simulink library "motorlib"  (R2018a)
settings: Solver=VariableStepAuto  StartTime=0.0  StopTime=10.0  RelTol=1e-3
libraries: $bdroot x5, aerolibatmos2 x4
settings Model: Creator=mairon  LastModifiedBy=mairon

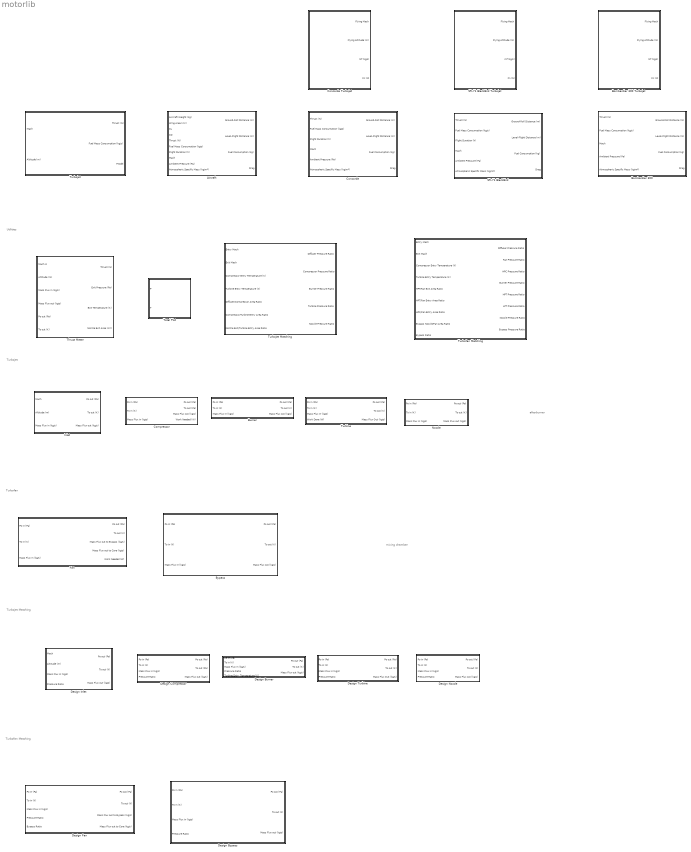
== system motorlib ==
  note: Turbofan Matching
  note: Utilities
  note: afterburner
  note: mixing chamber
  note: Turbofan
  note: Turbojet Matching
  note: Turbojet
  Aircraft : Subsystem
  Bombardier 300 : Subsystem  AncestorBlock=motorlib/Concorde
  Bombardier 300 Turbojet : Subsystem  AncestorBlock=motorlib/Concorde Turbojet
  Burner : Subsystem
  Bypass : Subsystem
  Compressor : Subsystem
  Concorde : Subsystem  AncestorBlock=motorlib/Aircraft
  Concorde Turbojet : Subsystem
  Design Burner : Subsystem  AncestorBlock=motorlib/Burner
  Design Bypass : Subsystem  AncestorBlock=motorlib/Bypass
  Design Compressor : Subsystem  AncestorBlock=motorlib/Compressor
  Design Fan : Subsystem  AncestorBlock=motorlib/Fan
  Design Inlet : Subsystem  AncestorBlock=motorlib/Inlet
  Design Nozzle : Subsystem  AncestorBlock=motorlib/Nozzle
  Design Turbine : Subsystem  AncestorBlock=motorlib/Turbine
  Fan : Subsystem
  Inlet : Subsystem
  Nozzle : Subsystem
  SR-71 BlackBird : Subsystem  AncestorBlock=motorlib/Concorde
  SR-71 BlackBird Turbojet : Subsystem  AncestorBlock=motorlib/Concorde Turbojet
  Thrust Meter : Subsystem
  Total Plot : MATLAB Function  TreatAsAtomicUnit=on
  Turbine : Subsystem
  Turbofan Matching : Subsystem  AncestorBlock=motorlib/Turbojet Matching
  Turbojet : Subsystem
  Turbojet Matching : Subsystem

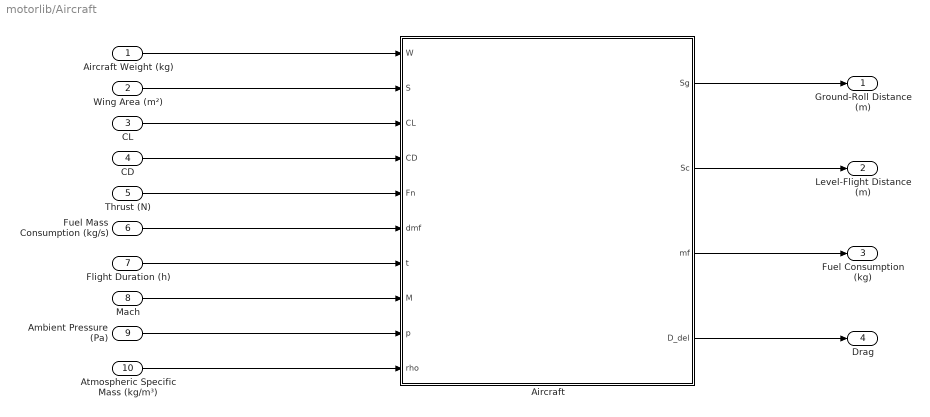
== system motorlib/Aircraft ==
  Aircraft Weight (kg) : Inport
  Wing Area (m²) : Inport  Port=2
  CL : Inport  Port=3
  CD : Inport  Port=4
  Thrust (N) : Inport  Port=5
  Fuel Mass Consumption (kg/s) : Inport  Port=6
  Flight Duration (h) : Inport  Port=7
  Mach : Inport  Port=8
  Ambient Pressure (Pa) : Inport  Port=9
  Atmospheric Specific Mass (kg/m³) : Inport  Port=10
  Aircraft : MATLAB Function  TreatAsAtomicUnit=on
  Ground-Roll Distance (m) : Outport
  Level-Flight Distance (m) : Outport  Port=2
  Fuel Consumption (kg) : Outport  Port=3
  Drag : Outport  Port=4
  wires:
  Aircraft/1(Sg) -> Ground-Roll Distance (m)/1
  Aircraft Weight (kg)/1 -> Aircraft/1(W)
  CD/1 -> Aircraft/4(CD)
  Wing Area (m²)/1 -> Aircraft/2(S)
  Aircraft/2(Sc) -> Level-Flight Distance (m)/1
  Ambient Pressure (Pa)/1 -> Aircraft/9(p)
  Fuel Mass Consumption (kg/s)/1 -> Aircraft/6(dmf)
  Aircraft/3(mf) -> Fuel Consumption (kg)/1
  Mach/1 -> Aircraft/8(M)
  CL/1 -> Aircraft/3(CL)
  Thrust (N)/1 -> Aircraft/5(Fn)
  Flight Duration (h)/1 -> Aircraft/7(t)
  Atmospheric Specific Mass (kg/m³)/1 -> Aircraft/10(rho)
  Aircraft/4(D_del) -> Drag/1

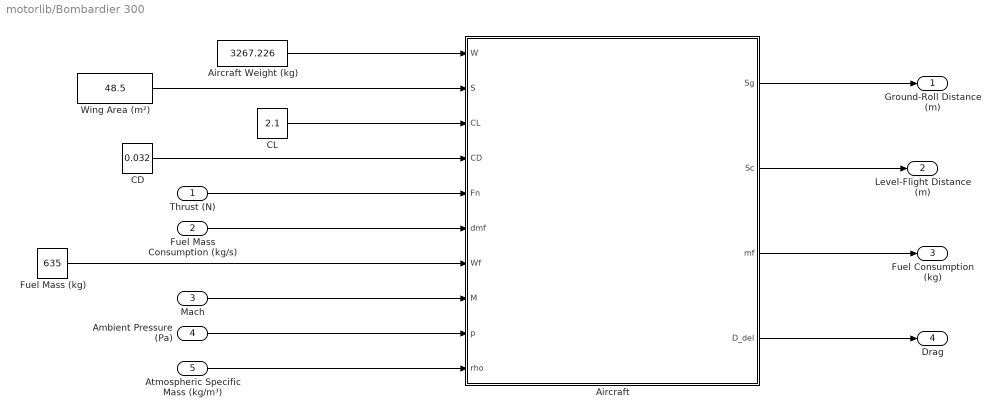
== system motorlib/Bombardier 300 ==
  Thrust (N) : Inport
  Fuel Mass Consumption (kg/s) : Inport  Port=2
  Mach : Inport  Port=3
  Ambient Pressure (Pa) : Inport  Port=4
  Atmospheric Specific Mass (kg/m³) : Inport  Port=5
  Aircraft : MATLAB Function  TreatAsAtomicUnit=on
  Aircraft Weight (kg) : Constant  Value=3267.226
  CD : Constant  Value=0.032
  CL : Constant  Value=2.1
  Fuel Mass (kg) : Constant  Value=635
  Wing Area (m²) : Constant  Value=48.5
  Ground-Roll Distance (m) : Outport
  Level-Flight Distance (m) : Outport  Port=2
  Fuel Consumption (kg) : Outport  Port=3
  Drag : Outport  Port=4
  wires:
  Aircraft/1(Sg) -> Ground-Roll Distance (m)/1
  Aircraft/2(Sc) -> Level-Flight Distance (m)/1
  Ambient Pressure (Pa)/1 -> Aircraft/9(p)
  Fuel Mass Consumption (kg/s)/1 -> Aircraft/6(dmf)
  Aircraft/3(mf) -> Fuel Consumption (kg)/1
  Mach/1 -> Aircraft/8(M)
  Thrust (N)/1 -> Aircraft/5(Fn)
  Fuel Mass (kg)/1 -> Aircraft/7(Wf)
  Atmospheric Specific Mass (kg/m³)/1 -> Aircraft/10(rho)
  Wing Area (m²)/1 -> Aircraft/2(S)
  CD/1 -> Aircraft/4(CD)
  CL/1 -> Aircraft/3(CL)
  Aircraft Weight (kg)/1 -> Aircraft/1(W)
  Aircraft/4(D_del) -> Drag/1

== system motorlib/Bombardier 300 Turbojet ==
  Altitude (m) : Constant  Value=9100
  Mach : Constant  Value=0.63
  Mass Fuel Consumption (kg/s) : Constant  Value=0.100
  Thrust (N) : Constant  Value=9319*2
  Flying Mach : Outport
  Flying Altitude (m) : Outport  Port=2
  mf (kg/s) : Outport  Port=3
  Fn (N) : Outport  Port=4
  wires:
  Altitude (m)/1 -> Flying Altitude (m)/1
  Mass Fuel Consumption (kg/s)/1 -> mf (kg/s)/1
  Mach/1 -> Flying Mach/1
  Thrust (N)/1 -> Fn (N)/1

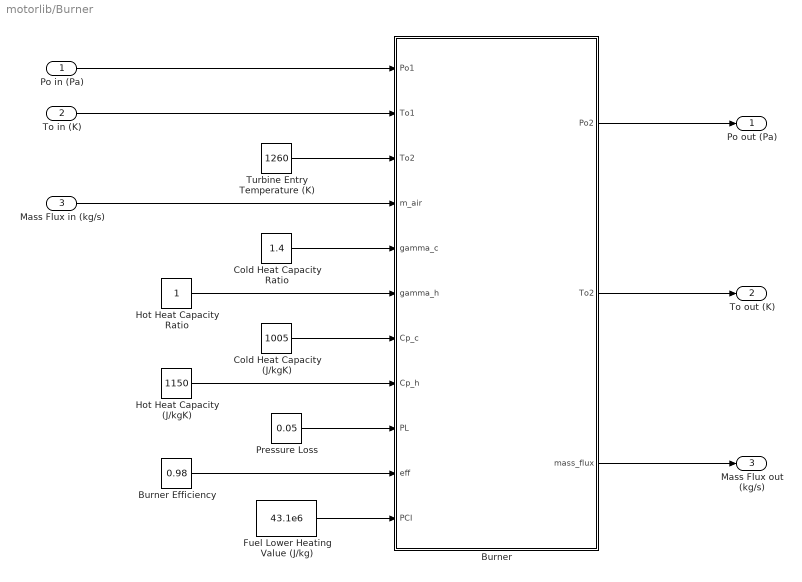
== system motorlib/Burner ==
  Po in (Pa) : Inport
  To in (K) : Inport  Port=2
  Mass Flux in (kg/s) : Inport  Port=3
  Burner : MATLAB Function  TreatAsAtomicUnit=on
  Burner Efficiency : Constant  Value=0.98
  Cold Heat Capacity (J/kgK) : Constant  Value=1005
  Cold Heat Capacity Ratio : Constant  Value=1.4
  Fuel Lower Heating Value (J/kg) : Constant  Value=43.1e6
  Hot Heat Capacity (J/kgK) : Constant  Value=1150
  Hot Heat Capacity Ratio : Constant
  Pressure Loss : Constant  Value=0.05
  Turbine Entry Temperature (K) : Constant  Value=1260
  Po out (Pa) : Outport
  To out (K) : Outport  Port=2
  Mass Flux out (kg/s) : Outport  Port=3
  wires:
  Cold Heat Capacity (J/kgK)/1 -> Burner/7(Cp_c)
  Pressure Loss/1 -> Burner/9(PL)
  Po in (Pa)/1 -> Burner/1(Po1)
  Burner/2(To2) -> To out (K)/1
  Turbine Entry Temperature (K)/1 -> Burner/3("To2 ")
  Hot Heat Capacity (J/kgK)/1 -> Burner/8(Cp_h)
  To in (K)/1 -> Burner/2(To1)
  Burner/3(mass_flux) -> Mass Flux out (kg/s)/1
  Fuel Lower Heating Value (J/kg)/1 -> Burner/11(PCI)
  Cold Heat Capacity Ratio/1 -> Burner/5(gamma_c)
  Mass Flux in (kg/s)/1 -> Burner/4(m_air)
  Burner/1(Po2) -> Po out (Pa)/1
  Burner Efficiency/1 -> Burner/10(eff)
  Hot Heat Capacity Ratio/1 -> Burner/6(gamma_h)

== system motorlib/Bypass ==
  Po in (Pa) : Inport
  To in (K) : Inport  Port=2
  Mass Flux in (kg/s) : Inport  Port=3
  Bypass : MATLAB Function  TreatAsAtomicUnit=on
  Heat Capacity Ratio : Constant  Value=1.4
  Pressure Loss : Constant  Value=0.05
  Po out (Pa) : Outport
  To out (K) : Outport  Port=2
  Mass Flux out (kg/s) : Outport  Port=3
  wires:
  Bypass/2(To2) -> To out (K)/1
  Bypass/1(Po2) -> Po out (Pa)/1
  Mass Flux in (kg/s)/1 -> Bypass/3("mass_flux ")
  To in (K)/1 -> Bypass/2(To1)
  Po in (Pa)/1 -> Bypass/1(Po1)
  Pressure Loss/1 -> Bypass/5(PL)
  Bypass/3(mass_flux) -> Mass Flux out (kg/s)/1
  Heat Capacity Ratio/1 -> Bypass/4(gamma)

== system motorlib/Compressor ==
  Po in (Pa) : Inport
  To in (K) : Inport  Port=2
  Mass Flux in (kg/s) : Inport  Port=3
  Compressor : MATLAB Function  TreatAsAtomicUnit=on
  Compressor Eficiency : Constant  Value=0.85
  Heat Capacity (J/kgK) : Constant  Value=1005
  Heat Capacity Ratio : Constant  Value=1.4
  Pressure Ratio : Constant  Value=13.5
  Po out (Pa) : Outport
  To out (Pa) : Outport  Port=2
  Mass Flux out (kg/s) : Outport  Port=3
  Work Needed (W) : Outport  Port=4
  wires:
  Mass Flux in (kg/s)/1 -> Compressor/3(m_air)
  Compressor/4(W) -> Work Needed (W)/1
  Compressor/2(To2) -> To out (Pa)/1
  Po in (Pa)/1 -> Compressor/1(Po1)
  Compressor/1(Po2) -> Po out (Pa)/1
  To in (K)/1 -> Compressor/2(To1)
  Compressor/3(mass_flux) -> Mass Flux out (kg/s)/1
  Heat Capacity Ratio/1 -> Compressor/4(gamma)
  Heat Capacity (J/kgK)/1 -> Compressor/5(Cp)
  Pressure Ratio/1 -> Compressor/6(PR)
  Compressor Eficiency/1 -> Compressor/7(eff)

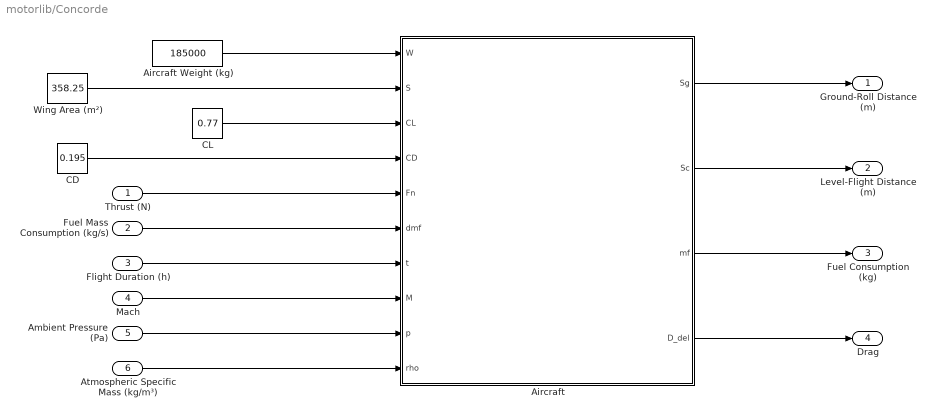
== system motorlib/Concorde ==
  Thrust (N) : Inport
  Fuel Mass Consumption (kg/s) : Inport  Port=2
  Flight Duration (h) : Inport  Port=3
  Mach : Inport  Port=4
  Ambient Pressure (Pa) : Inport  Port=5
  Atmospheric Specific Mass (kg/m³) : Inport  Port=6
  Aircraft : MATLAB Function  TreatAsAtomicUnit=on
  Aircraft Weight (kg) : Constant  Value=185000
  CD : Constant  Value=0.195
  CL : Constant  Value=0.77
  Wing Area (m²) : Constant  Value=358.25
  Ground-Roll Distance (m) : Outport
  Level-Flight Distance (m) : Outport  Port=2
  Fuel Consumption (kg) : Outport  Port=3
  Drag : Outport  Port=4
  wires:
  Aircraft/1(Sg) -> Ground-Roll Distance (m)/1
  Aircraft/2(Sc) -> Level-Flight Distance (m)/1
  Ambient Pressure (Pa)/1 -> Aircraft/9(p)
  Fuel Mass Consumption (kg/s)/1 -> Aircraft/6(dmf)
  Aircraft/3(mf) -> Fuel Consumption (kg)/1
  Mach/1 -> Aircraft/8(M)
  Thrust (N)/1 -> Aircraft/5(Fn)
  Flight Duration (h)/1 -> Aircraft/7(t)
  Atmospheric Specific Mass (kg/m³)/1 -> Aircraft/10(rho)
  Wing Area (m²)/1 -> Aircraft/2(S)
  CD/1 -> Aircraft/4(CD)
  CL/1 -> Aircraft/3(CL)
  Aircraft Weight (kg)/1 -> Aircraft/1(W)
  Aircraft/4(D_del) -> Drag/1

== system motorlib/Concorde Turbojet ==
  Altitude (m) : Constant  Value=18000
  Mach : Constant  Value=2
  Mass Fuel Consumption (kg/s) : Constant  Value=5.699
  Thrust (N) : Constant  Value=17233*4
  Flying Mach : Outport
  Flying Altitude (m) : Outport  Port=2
  mf (kg/s) : Outport  Port=3
  Fn (N) : Outport  Port=4
  wires:
  Thrust (N)/1 -> Fn (N)/1
  Mach/1 -> Flying Mach/1
  Mass Fuel Consumption (kg/s)/1 -> mf (kg/s)/1
  Altitude (m)/1 -> Flying Altitude (m)/1

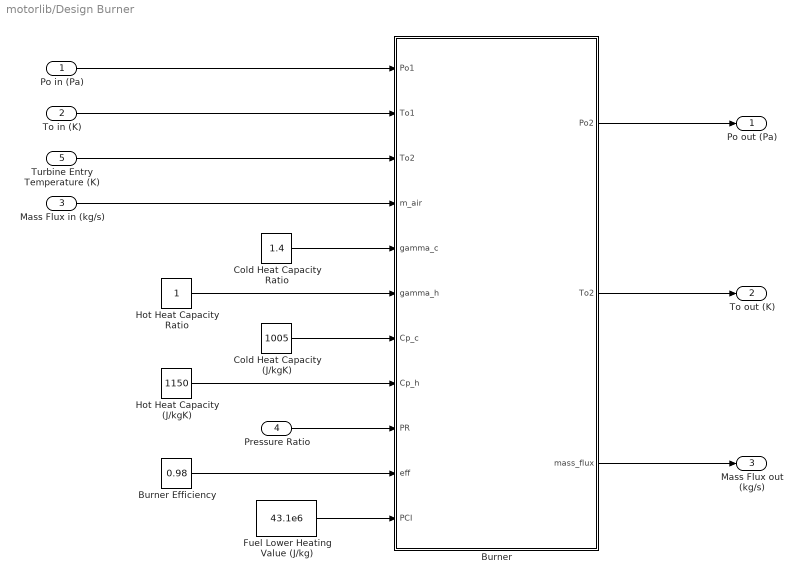
== system motorlib/Design Burner ==
  Po in (Pa) : Inport
  To in (K) : Inport  Port=2
  Mass Flux in (kg/s) : Inport  Port=3
  Pressure Ratio : Inport  Port=4
  Turbine Entry Temperature (K) : Inport  Port=5
  Burner : MATLAB Function  TreatAsAtomicUnit=on
  Burner Efficiency : Constant  Value=0.98
  Cold Heat Capacity (J/kgK) : Constant  Value=1005
  Cold Heat Capacity Ratio : Constant  Value=1.4
  Fuel Lower Heating Value (J/kg) : Constant  Value=43.1e6
  Hot Heat Capacity (J/kgK) : Constant  Value=1150
  Hot Heat Capacity Ratio : Constant
  Po out (Pa) : Outport
  To out (K) : Outport  Port=2
  Mass Flux out (kg/s) : Outport  Port=3
  wires:
  Hot Heat Capacity Ratio/1 -> Burner/6(gamma_h)
  Burner Efficiency/1 -> Burner/10(eff)
  Burner/1(Po2) -> Po out (Pa)/1
  Mass Flux in (kg/s)/1 -> Burner/4(m_air)
  Cold Heat Capacity Ratio/1 -> Burner/5(gamma_c)
  Fuel Lower Heating Value (J/kg)/1 -> Burner/11(PCI)
  Burner/3(mass_flux) -> Mass Flux out (kg/s)/1
  To in (K)/1 -> Burner/2(To1)
  Hot Heat Capacity (J/kgK)/1 -> Burner/8(Cp_h)
  Turbine Entry Temperature (K)/1 -> Burner/3("To2 ")
  Burner/2(To2) -> To out (K)/1
  Po in (Pa)/1 -> Burner/1(Po1)
  Pressure Ratio/1 -> Burner/9(PR)
  Cold Heat Capacity (J/kgK)/1 -> Burner/7(Cp_c)

== system motorlib/Design Bypass ==
  Po in (Pa) : Inport
  To in (K) : Inport  Port=2
  Mass Flux in (kg/s) : Inport  Port=3
  Pressure Ratio : Inport  Port=4
  Bypass : MATLAB Function  TreatAsAtomicUnit=on
  Heat Capacity Ratio : Constant  Value=1.4
  Po out (Pa) : Outport
  To out (K) : Outport  Port=2
  Mass Flux out (kg/s) : Outport  Port=3
  wires:
  Bypass/2(To2) -> To out (K)/1
  Bypass/1(Po2) -> Po out (Pa)/1
  Mass Flux in (kg/s)/1 -> Bypass/3("mass_flux ")
  To in (K)/1 -> Bypass/2(To1)
  Po in (Pa)/1 -> Bypass/1(Po1)
  Pressure Ratio/1 -> Bypass/5(PR)
  Bypass/3(mass_flux) -> Mass Flux out (kg/s)/1
  Heat Capacity Ratio/1 -> Bypass/4(gamma)

== system motorlib/Design Compressor ==
  Po in (Pa) : Inport
  To in (K) : Inport  Port=2
  Mass Flux in (kg/s) : Inport  Port=3
  Pressure Ratio : Inport  Port=4
  Compressor : MATLAB Function  TreatAsAtomicUnit=on
  Compressor Eficiency : Constant  Value=0.85
  Heat Capacity (J/kgK) : Constant  Value=1005
  Heat Capacity Ratio : Constant  Value=1.4
  Po out (Pa) : Outport
  To out (Pa) : Outport  Port=2
  Mass Flux out (kg/s) : Outport  Port=3
  wires:
  Compressor Eficiency/1 -> Compressor/7(eff)
  Pressure Ratio/1 -> Compressor/6(PR)
  Heat Capacity (J/kgK)/1 -> Compressor/5(Cp)
  Heat Capacity Ratio/1 -> Compressor/4(gamma)
  Compressor/3(mass_flux) -> Mass Flux out (kg/s)/1
  To in (K)/1 -> Compressor/2(To1)
  Compressor/1(Po2) -> Po out (Pa)/1
  Po in (Pa)/1 -> Compressor/1(Po1)
  Compressor/2(To2) -> To out (Pa)/1
  Mass Flux in (kg/s)/1 -> Compressor/3(m_air)

== system motorlib/Design Fan ==
  Po in (Pa) : Inport
  To in (K) : Inport  Port=2
  Mass Flux in (kg/s) : Inport  Port=3
  Pressure Ratio : Inport  Port=4
  Bypass Ratio : Inport  Port=5
  Efficiency : Constant  Value=0.84
  Fan : MATLAB Function  TreatAsAtomicUnit=on
  Heat Capacity (J/kgK) : Constant  Value=1005
  Heat Capacity Ratio : Constant  Value=1.4
  Po out (Pa) : Outport
  To out (K) : Outport  Port=2
  Mass Flux out to Bypass (kg/s) : Outport  Port=3
  Mass Flux out to Core (kg/s) : Outport  Port=4
  wires:
  Fan/1(Po2) -> Po out (Pa)/1
  Po in (Pa)/1 -> Fan/1(Po1)
  Fan/2(To2) -> To out (K)/1
  Heat Capacity (J/kgK)/1 -> Fan/5(Cp)
  Fan/4(mass_flux_core) -> Mass Flux out to Core (kg/s)/1
  Fan/3(mass_flux_bp) -> Mass Flux out to Bypass (kg/s)/1
  Efficiency/1 -> Fan/7(eff)
  Heat Capacity Ratio/1 -> Fan/4(gamma)
  To in (K)/1 -> Fan/2(To1)
  Bypass Ratio/1 -> Fan/8(B)
  Mass Flux in (kg/s)/1 -> Fan/3(mass_flux)
  Pressure Ratio/1 -> Fan/6(PR)

== system motorlib/Design Inlet ==
  Mach : Inport
  Altitude (m) : Inport  Port=2
  Mass Flux in (kg/s) : Inport  Port=3
  Pressure Ratio : Inport  Port=4
  Heat Capacity Ratio : Constant  Value=1.4
  ISA Atmosphere Model : aerolibatmos2/ISA Atmosphere Model  custom=off  g=9.80665  gamma=1.4  R=287.0531  L=0.0065  h_trop=11000  h_strat=20000  rho0=1.225  P0=101325  T0=288.15  h0=0
      settings: SourceProductName=Aerospace Blockset
  Inlet : MATLAB Function  TreatAsAtomicUnit=on
  Po out (Pa) : Outport
  To out (K) : Outport  Port=2
  Mass Flux out (kg/s) : Outport  Port=3
  wires:
  Heat Capacity Ratio/1 -> Inlet/4(gamma)
  Inlet/3(mass_flux) -> Mass Flux out (kg/s)/1
  Mass Flux in (kg/s)/1 -> Inlet/6(m_air)
  Altitude (m)/1 -> ISA Atmosphere Model/1
  ISA Atmosphere Model/3 -> Inlet/2(P)
  Pressure Ratio/1 -> Inlet/5(PR)
  Inlet/1(Po) -> Po out (Pa)/1
  ISA Atmosphere Model/1 -> Inlet/3(T)
  Mach/1 -> Inlet/1(Mach)
  Inlet/2(To) -> To out (K)/1

== system motorlib/Design Nozzle ==
  Po in (Pa) : Inport
  To in (K) : Inport  Port=2
  Mass Flux in (kg/s) : Inport  Port=3
  Pressure Ratio : Inport  Port=4
  Hot Heat Capacity Ratio : Constant  Value=1.333
  Nozzle : MATLAB Function  TreatAsAtomicUnit=on
  Po out (Pa) : Outport
  To out (K) : Outport  Port=2
  Mass Flux out (kg/s) : Outport  Port=3
  wires:
  Hot Heat Capacity Ratio/1 -> Nozzle/4(gamma)
  Pressure Ratio/1 -> Nozzle/5(PR)
  Nozzle/3(mass_flux) -> Mass Flux out (kg/s)/1
  Nozzle/1(Po2) -> Po out (Pa)/1
  Mass Flux in (kg/s)/1 -> Nozzle/3("mass_flux ")
  To in (K)/1 -> Nozzle/2(To1)
  Nozzle/2(To2) -> To out (K)/1
  Po in (Pa)/1 -> Nozzle/1(Po1)

== system motorlib/Design Turbine ==
  Po in (Pa) : Inport
  To in (K) : Inport  Port=2
  Mass Flux in (kg/s) : Inport  Port=3
  Pressure Ratio : Inport  Port=4
  Efficiency : Constant
  Hot Heat Capacity Ratio : Constant  Value=1.333
  Turbine : MATLAB Function  TreatAsAtomicUnit=on
  Po out (Pa) : Outport
  To out (K) : Outport  Port=2
  Mass Flux Out (kg/s) : Outport  Port=3
  wires:
  Mass Flux in (kg/s)/1 -> Turbine/3("mass_flux ")
  Po in (Pa)/1 -> Turbine/1(Po1)
  Turbine/3(mass_flux) -> Mass Flux Out (kg/s)/1
  Hot Heat Capacity Ratio/1 -> Turbine/5(gamma)
  Turbine/1(Po2) -> Po out (Pa)/1
  Pressure Ratio/1 -> Turbine/4(PR)
  To in (K)/1 -> Turbine/2(To1)
  Turbine/2(To2) -> To out (K)/1
  Efficiency/1 -> Turbine/6(eff)

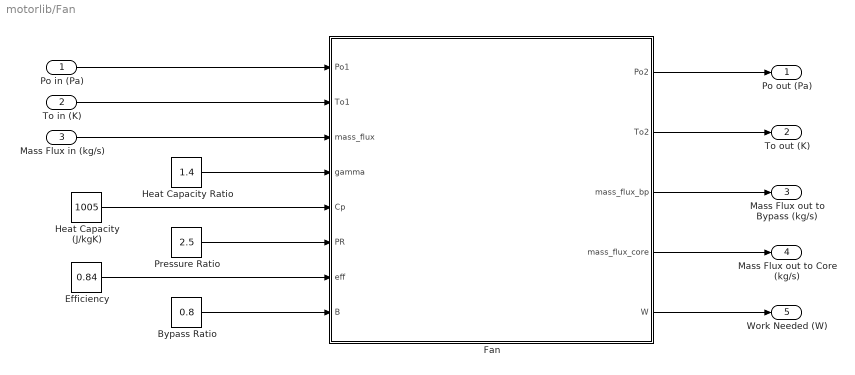
== system motorlib/Fan ==
  Po in (Pa) : Inport
  To in (K) : Inport  Port=2
  Mass Flux in (kg/s) : Inport  Port=3
  Bypass Ratio : Constant  Value=0.8
  Efficiency : Constant  Value=0.84
  Fan : MATLAB Function  TreatAsAtomicUnit=on
  Heat Capacity (J/kgK) : Constant  Value=1005
  Heat Capacity Ratio : Constant  Value=1.4
  Pressure Ratio : Constant  Value=2.5
  Po out (Pa) : Outport
  To out (K) : Outport  Port=2
  Mass Flux out to Bypass (kg/s) : Outport  Port=3
  Mass Flux out to Core (kg/s) : Outport  Port=4
  Work Needed (W) : Outport  Port=5
  wires:
  Fan/1(Po2) -> Po out (Pa)/1
  Po in (Pa)/1 -> Fan/1(Po1)
  Fan/2(To2) -> To out (K)/1
  Heat Capacity (J/kgK)/1 -> Fan/5(Cp)
  Fan/4(mass_flux_core) -> Mass Flux out to Core (kg/s)/1
  Fan/5(W) -> Work Needed (W)/1
  Fan/3(mass_flux_bp) -> Mass Flux out to Bypass (kg/s)/1
  Efficiency/1 -> Fan/7(eff)
  Heat Capacity Ratio/1 -> Fan/4(gamma)
  To in (K)/1 -> Fan/2(To1)
  Bypass Ratio/1 -> Fan/8(B)
  Mass Flux in (kg/s)/1 -> Fan/3(mass_flux)
  Pressure Ratio/1 -> Fan/6(PR)

== system motorlib/Inlet ==
  Mach : Inport
  Altitude (m) : Inport  Port=2
  Mass Flux in (kg/s) : Inport  Port=3
  Heat Capacity Ratio : Constant  Value=1.4
  ISA Atmosphere Model : aerolibatmos2/ISA Atmosphere Model  custom=off  g=9.80665  gamma=1.4  R=287.0531  L=0.0065  h_trop=11000  h_strat=20000  rho0=1.225  P0=101325  T0=288.15  h0=0
      settings: SourceProductName=Aerospace Blockset
  Inlet : MATLAB Function  TreatAsAtomicUnit=on
  Pressure Loss : Constant  Value=0
  Po out (Pa) : Outport
  To out (K) : Outport  Port=2
  Mass Flux out (kg/s) : Outport  Port=3
  wires:
  Inlet/2(To) -> To out (K)/1
  Mach/1 -> Inlet/1(Mach)
  ISA Atmosphere Model/1 -> Inlet/3(T)
  Inlet/1(Po) -> Po out (Pa)/1
  Pressure Loss/1 -> Inlet/5(PL)
  ISA Atmosphere Model/3 -> Inlet/2(P)
  Altitude (m)/1 -> ISA Atmosphere Model/1
  Mass Flux in (kg/s)/1 -> Inlet/6(m_air)
  Inlet/3(mass_flux) -> Mass Flux out (kg/s)/1
  Heat Capacity Ratio/1 -> Inlet/4(gamma)

== system motorlib/Nozzle ==
  Po in (Pa) : Inport
  To in (K) : Inport  Port=2
  Mass Flux in (kg/s) : Inport  Port=3
  Hot Heat Capacity Ratio : Constant  Value=1.333
  Nozzle : MATLAB Function  TreatAsAtomicUnit=on
  Pressure Loss : Constant  Value=0.02
  Po out (Pa) : Outport
  To out (K) : Outport  Port=2
  Mass Flux out (kg/s) : Outport  Port=3
  wires:
  Po in (Pa)/1 -> Nozzle/1(Po1)
  Nozzle/2(To2) -> To out (K)/1
  To in (K)/1 -> Nozzle/2(To1)
  Mass Flux in (kg/s)/1 -> Nozzle/3("mass_flux ")
  Nozzle/1(Po2) -> Po out (Pa)/1
  Nozzle/3(mass_flux) -> Mass Flux out (kg/s)/1
  Pressure Loss/1 -> Nozzle/5(PL)
  Hot Heat Capacity Ratio/1 -> Nozzle/4(gamma)

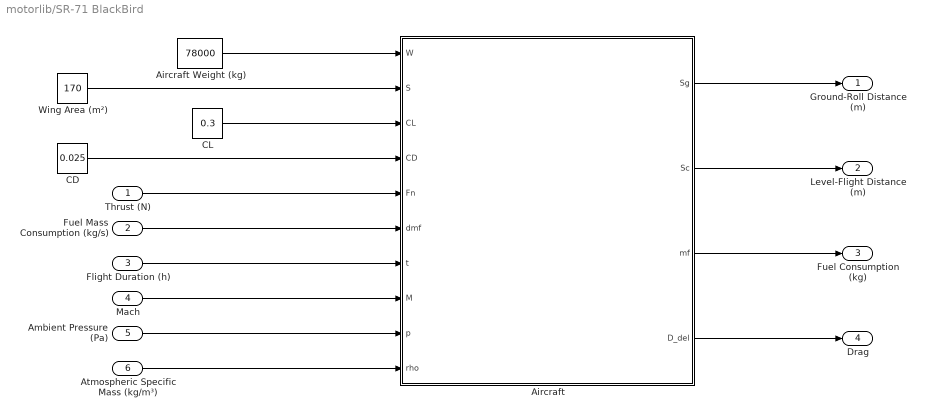
== system motorlib/SR-71 BlackBird ==
  Thrust (N) : Inport
  Fuel Mass Consumption (kg/s) : Inport  Port=2
  Flight Duration (h) : Inport  Port=3
  Mach : Inport  Port=4
  Ambient Pressure (Pa) : Inport  Port=5
  Atmospheric Specific Mass (kg/m³) : Inport  Port=6
  Aircraft : MATLAB Function  TreatAsAtomicUnit=on
  Aircraft Weight (kg) : Constant  Value=78000
  CD : Constant  Value=0.025
  CL : Constant  Value=0.3
  Wing Area (m²) : Constant  Value=170
  Ground-Roll Distance (m) : Outport
  Level-Flight Distance (m) : Outport  Port=2
  Fuel Consumption (kg) : Outport  Port=3
  Drag : Outport  Port=4
  wires:
  Aircraft/1(Sg) -> Ground-Roll Distance (m)/1
  Aircraft/2(Sc) -> Level-Flight Distance (m)/1
  Ambient Pressure (Pa)/1 -> Aircraft/9(p)
  Fuel Mass Consumption (kg/s)/1 -> Aircraft/6(dmf)
  Aircraft/3(mf) -> Fuel Consumption (kg)/1
  Mach/1 -> Aircraft/8(M)
  Thrust (N)/1 -> Aircraft/5(Fn)
  Flight Duration (h)/1 -> Aircraft/7(t)
  Atmospheric Specific Mass (kg/m³)/1 -> Aircraft/10(rho)
  Wing Area (m²)/1 -> Aircraft/2(S)
  CD/1 -> Aircraft/4(CD)
  CL/1 -> Aircraft/3(CL)
  Aircraft Weight (kg)/1 -> Aircraft/1(W)
  Aircraft/4(D_del) -> Drag/1

== system motorlib/SR-71 BlackBird Turbojet ==
  Altitude (m) : Constant  Value=25910
  Mach : Constant  Value=3.17
  Mass Fuel Consumption (kg/s) : Constant  Value=4.17
  Thrust (N) : Constant  Value=151000*2
  Flying Mach : Outport
  Flying Altitude (m) : Outport  Port=2
  mf (kg/s) : Outport  Port=3
  Fn (N) : Outport  Port=4
  wires:
  Thrust (N)/1 -> Fn (N)/1
  Mach/1 -> Flying Mach/1
  Mass Fuel Consumption (kg/s)/1 -> mf (kg/s)/1
  Altitude (m)/1 -> Flying Altitude (m)/1

== system motorlib/Thrust Meter ==
  Mach in : Inport
  Altitude (m) : Inport  Port=2
  Mass Flux in (kg/s) : Inport  Port=3
  Mass Flux out (kg/s) : Inport  Port=4
  Po out (Pa) : Inport  Port=5
  To out (K) : Inport  Port=6
  Hot Heat Capacity Ratio : Constant  Value=1.333
  ISA Atmosphere Model1 : aerolibatmos2/ISA Atmosphere Model  custom=off  g=9.80665  gamma=1.4  R=287.0531  L=0.0065  h_trop=11000  h_strat=20000  rho0=1.225  P0=101325  T0=288.15  h0=0
      settings: SourceProductName=Aerospace Blockset
  Thrust : MATLAB Function  TreatAsAtomicUnit=on
  Thrust (N) : Outport
  Exit Pressure (Pa) : Outport  Port=2
  Exit Temperature (K) : Outport  Port=3
  Nozzle Exit Area (m²) : Outport  Port=4
  wires:
  ISA Atmosphere Model1/1 -> Thrust/4(Tatm)
  ISA Atmosphere Model1/3 -> Thrust/3(Patm)
  Altitude (m)/1 -> ISA Atmosphere Model1/1
  Mach in/1 -> Thrust/1(Mo)
  ISA Atmosphere Model1/2 -> Thrust/2(a)
  Mass Flux in (kg/s)/1 -> Thrust/5(mass_flux_0)
  Mass Flux out (kg/s)/1 -> Thrust/6(mass_flux)
  Hot Heat Capacity Ratio/1 -> Thrust/9(gamma_h)
  Po out (Pa)/1 -> Thrust/7(Po2)
  To out (K)/1 -> Thrust/8(To2)
  Thrust/2(Pe) -> Exit Pressure (Pa)/1
  Thrust/3(Te) -> Exit Temperature (K)/1
  Thrust/1(FN) -> Thrust (N)/1
  Thrust/4(Ae) -> Nozzle Exit Area (m²)/1

== system motorlib/Turbine ==
  Po in (Pa) : Inport
  To in (K) : Inport  Port=2
  Mass Flux in (kg/s) : Inport  Port=3
  Work Done (W) : Inport  Port=4
  Hot Heat Capacity (J/kgK) : Constant  Value=1150
  Hot Heat Capacity Ratio : Constant  Value=1.333
  Turbine : MATLAB Function  TreatAsAtomicUnit=on
  Turbine Efficiency : Constant  Value=0.92
  Po out (Pa) : Outport
  To out (K) : Outport  Port=2
  Mass Flux Out (kg/s) : Outport  Port=3
  wires:
  Turbine/2(To2) -> To out (K)/1
  To in (K)/1 -> Turbine/2(To1)
  Work Done (W)/1 -> Turbine/4(W)
  Turbine/1(Po2) -> Po out (Pa)/1
  Hot Heat Capacity (J/kgK)/1 -> Turbine/6(Cp_h)
  Hot Heat Capacity Ratio/1 -> Turbine/5(gamma_h)
  Turbine/3(mass_flux) -> Mass Flux Out (kg/s)/1
  Turbine Efficiency/1 -> Turbine/7(eff)
  Po in (Pa)/1 -> Turbine/1(Po1)
  Mass Flux in (kg/s)/1 -> Turbine/3("mass_flux ")

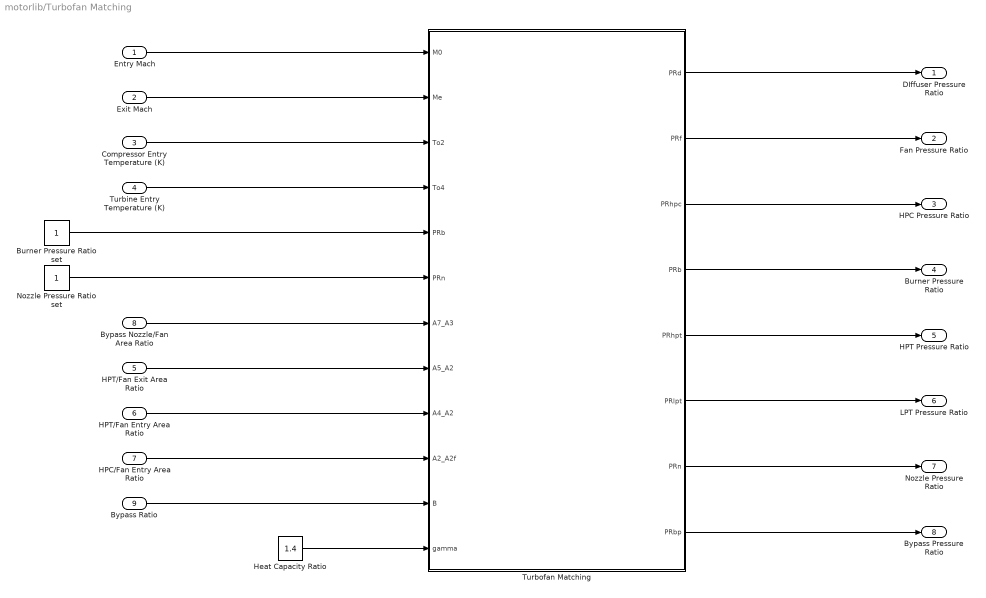
== system motorlib/Turbofan Matching ==
  Entry Mach : Inport
  Exit Mach : Inport  Port=2
  Compressor Entry Temperature (K) : Inport  Port=3
  Turbine Entry Temperature (K) : Inport  Port=4
  HPT/Fan Exit Area Ratio : Inport  Port=5
  HPT/Fan Entry Area Ratio : Inport  Port=6
  HPC/Fan Entry Area Ratio : Inport  Port=7
  Bypass Nozzle/Fan Area Ratio : Inport  Port=8
  "Bypass Ratio " : Inport  Port=9
  Burner Pressure Ratio set : Constant
  Heat Capacity Ratio : Constant  Value=1.4
  Nozzle Pressure Ratio set : Constant
  Turbofan Matching : MATLAB Function  TreatAsAtomicUnit=on
  DIffuser Pressure Ratio : Outport
  Fan Pressure Ratio : Outport  Port=2
  HPC Pressure Ratio : Outport  Port=3
  Burner Pressure Ratio : Outport  Port=4
  HPT Pressure Ratio : Outport  Port=5
  LPT Pressure Ratio : Outport  Port=6
  Nozzle Pressure Ratio : Outport  Port=7
  Bypass Pressure Ratio : Outport  Port=8
  wires:
  Burner Pressure Ratio set/1 -> Turbofan Matching/5("PRb ")
  Nozzle Pressure Ratio set/1 -> Turbofan Matching/6("PRn ")
  Turbofan Matching/1(PRd) -> DIffuser Pressure Ratio/1
  Entry Mach/1 -> Turbofan Matching/1(M0)
  Turbofan Matching/3(PRhpc) -> HPC Pressure Ratio/1
  HPC/Fan Entry Area Ratio/1 -> Turbofan Matching/10(A2_A2f)
  Turbine Entry Temperature (K)/1 -> Turbofan Matching/4(To4)
  Heat Capacity Ratio/1 -> Turbofan Matching/12(gamma)
  Exit Mach/1 -> Turbofan Matching/2(Me)
  Turbofan Matching/4(PRb) -> Burner Pressure Ratio/1
  HPT/Fan Entry Area Ratio/1 -> Turbofan Matching/9(A4_A2)
  Turbofan Matching/7(PRn) -> Nozzle Pressure Ratio/1
  Turbofan Matching/2(PRf) -> Fan Pressure Ratio/1
  Compressor Entry Temperature (K)/1 -> Turbofan Matching/3(To2)
  HPT/Fan Exit Area Ratio/1 -> Turbofan Matching/8(A5_A2)
  Bypass Nozzle/Fan Area Ratio/1 -> Turbofan Matching/7(A7_A3)
  "Bypass Ratio "/1 -> Turbofan Matching/11(B)
  Turbofan Matching/5(PRhpt) -> HPT Pressure Ratio/1
  Turbofan Matching/6(PRlpt) -> LPT Pressure Ratio/1
  Turbofan Matching/8(PRbp) -> Bypass Pressure Ratio/1

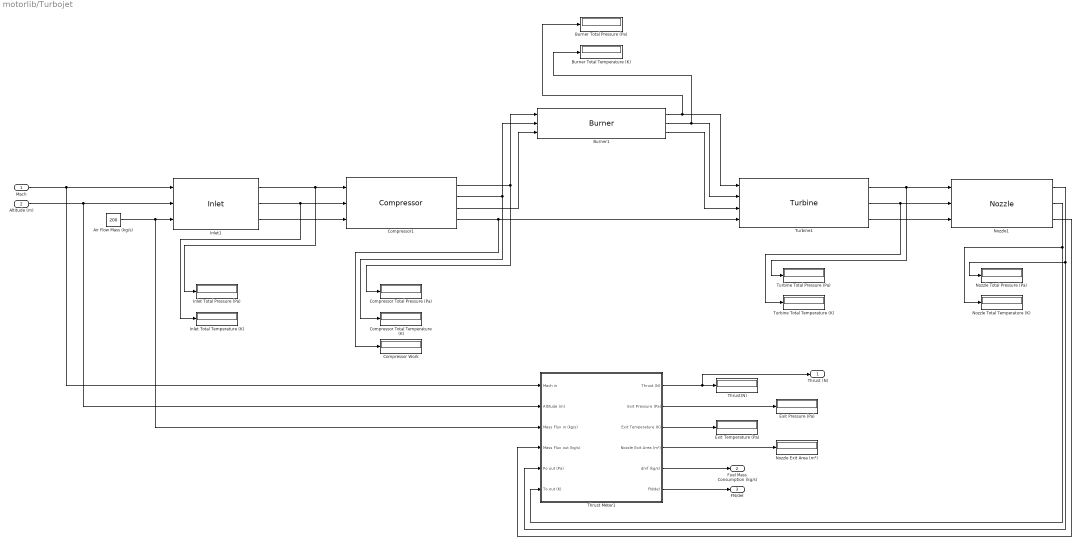
== system motorlib/Turbojet ==
  Mach : Inport
  Altitude (m) : Inport  Port=2
  Air Flow Mass (kg/s) : Constant  Value=200
  Burner Total Pressure (Pa) : Display
  Burner Total Temperature (K) : Display
  Burner1 : $bdroot/Burner
  Compressor Total Pressure (Pa) : Display
  Compressor Total Temperature (K) : Display
  Compressor Work : Display
  Compressor1 : $bdroot/Compressor
  Exit Pressure (Pa) : Display
  Exit Temperature (Pa) : Display
  Inlet Total Pressure (Pa) : Display
  Inlet Total Temperature (K) : Display
  Inlet1 : $bdroot/Inlet
  Nozzle Exit Area (m²) : Display
  "Nozzle Total Pressure (Pa) " : Display
  Nozzle Total Temperature (K) : Display
  Nozzle1 : $bdroot/Nozzle
  Thrust Meter1 : Subsystem  AncestorBlock=motorlib/Thrust Meter
  Thrust(N) : Display
  Turbine Total Pressure (Pa) : Display
  Turbine Total Temperature (K) : Display
  Turbine1 : $bdroot/Turbine
  Thrust (N) : Outport
  Fuel Mass Consumption (kg/s) : Outport  Port=2
  FN/del : Outport  Port=3
  wires:
  Thrust Meter1/4(Nozzle Exit Area (m²)) -> Nozzle Exit Area (m²)/1
  Mach/1 -> Inlet1/1, Thrust Meter1/1(Mach in)
  Turbine1/2 -> Turbine Total Temperature (K)/1, Nozzle1/2
  Burner1/1 -> Turbine1/1, Burner Total Pressure (Pa)/1
  Turbine1/1 -> Nozzle1/1, Turbine Total Pressure (Pa)/1
  Burner1/2 -> Turbine1/2, Burner Total Temperature (K)/1
  Turbine1/3 -> Nozzle1/3
  Thrust Meter1/3(Exit Temperature (K)) -> Exit Temperature (Pa)/1
  Nozzle1/2 -> Thrust Meter1/6(To out (K)), Nozzle Total Temperature (K)/1
  Nozzle1/1 -> Thrust Meter1/5(Po out (Pa)), "Nozzle Total Pressure (Pa) "/1
  Inlet1/2 -> Inlet Total Temperature (K)/1, Compressor1/2
  Inlet1/1 -> Inlet Total Pressure (Pa)/1, Compressor1/1
  Compressor1/1 -> Burner1/1, Compressor Total Pressure (Pa)/1
  Altitude (m)/1 -> Inlet1/2, Thrust Meter1/2(Altitude (m))
  Compressor1/2 -> Burner1/2, Compressor Total Temperature (K)/1
  Compressor1/4 -> Compressor Work/1, Turbine1/4
  Thrust Meter1/1(Thrust (N)) -> Thrust (N)/1, Thrust(N)/1
  Air Flow Mass (kg/s)/1 -> Thrust Meter1/3(Mass Flux in (kg/s)), Inlet1/3
  Burner1/3 -> Turbine1/3
  Compressor1/3 -> Burner1/3
  Thrust Meter1/2(Exit Pressure (Pa)) -> Exit Pressure (Pa)/1
  Inlet1/3 -> Compressor1/3
  Nozzle1/3 -> Thrust Meter1/4(Mass Flux out (kg/s))
  Thrust Meter1/5(dmf (kg/s)) -> Fuel Mass Consumption (kg/s)/1
  Thrust Meter1/6(FN/del) -> FN/del/1

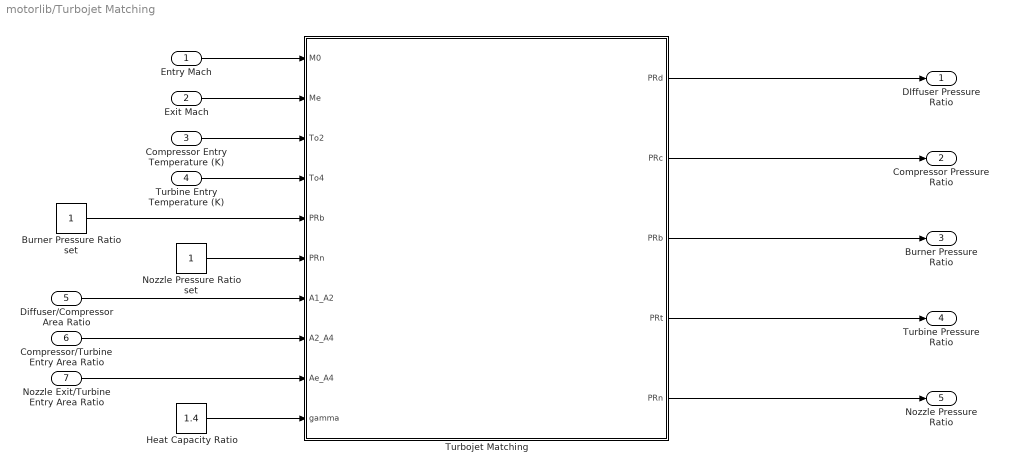
== system motorlib/Turbojet Matching ==
  Entry Mach : Inport
  Exit Mach : Inport  Port=2
  Compressor Entry Temperature (K) : Inport  Port=3
  Turbine Entry Temperature (K) : Inport  Port=4
  Diffuser/Compressor Area Ratio : Inport  Port=5
  Compressor/Turbine Entry Area Ratio : Inport  Port=6
  Nozzle Exit/Turbine Entry Area Ratio : Inport  Port=7
  Burner Pressure Ratio set : Constant
  Heat Capacity Ratio : Constant  Value=1.4
  Nozzle Pressure Ratio set : Constant
  Turbojet Matching : MATLAB Function  TreatAsAtomicUnit=on
  DIffuser Pressure Ratio : Outport
  Compressor Pressure Ratio : Outport  Port=2
  Burner Pressure Ratio : Outport  Port=3
  Turbine Pressure Ratio : Outport  Port=4
  Nozzle Pressure Ratio : Outport  Port=5
  wires:
  Burner Pressure Ratio set/1 -> Turbojet Matching/5("PRb ")
  Nozzle Pressure Ratio set/1 -> Turbojet Matching/6("PRn ")
  Turbojet Matching/1(PRd) -> DIffuser Pressure Ratio/1
  Entry Mach/1 -> Turbojet Matching/1(M0)
  Turbojet Matching/4(PRt) -> Turbine Pressure Ratio/1
  Nozzle Exit/Turbine Entry Area Ratio/1 -> Turbojet Matching/9(Ae_A4)
  Turbine Entry Temperature (K)/1 -> Turbojet Matching/4(To4)
  Heat Capacity Ratio/1 -> Turbojet Matching/10(gamma)
  Exit Mach/1 -> Turbojet Matching/2(Me)
  Turbojet Matching/3(PRb) -> Burner Pressure Ratio/1
  Compressor/Turbine Entry Area Ratio/1 -> Turbojet Matching/8(A2_A4)
  Turbojet Matching/5(PRn) -> Nozzle Pressure Ratio/1
  Turbojet Matching/2(PRc) -> Compressor Pressure Ratio/1
  Compressor Entry Temperature (K)/1 -> Turbojet Matching/3(To2)
  Diffuser/Compressor Area Ratio/1 -> Turbojet Matching/7(A1_A2)

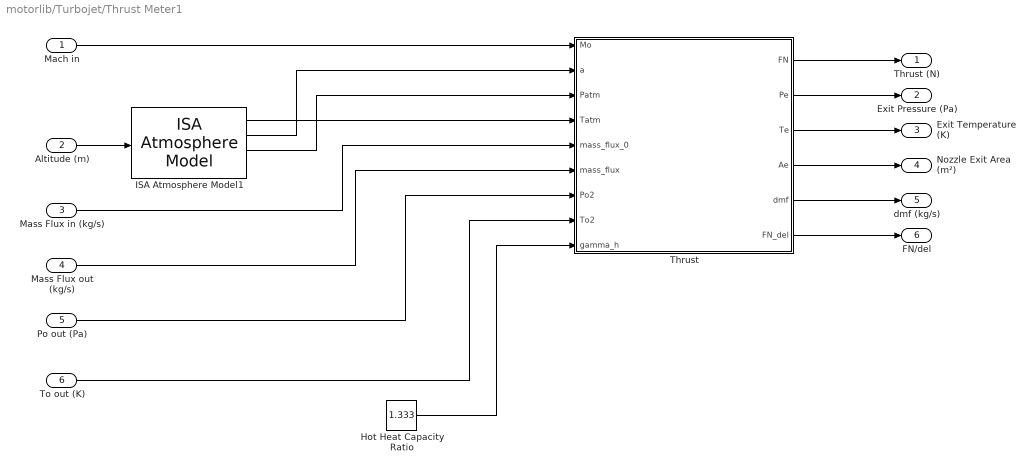
== system motorlib/Turbojet/Thrust Meter1 ==
  Mach in : Inport
  Altitude (m) : Inport  Port=2
  Mass Flux in (kg/s) : Inport  Port=3
  Mass Flux out (kg/s) : Inport  Port=4
  Po out (Pa) : Inport  Port=5
  To out (K) : Inport  Port=6
  Hot Heat Capacity Ratio : Constant  Value=1.333
  ISA Atmosphere Model1 : aerolibatmos2/ISA Atmosphere Model  custom=off  g=9.80665  gamma=1.4  R=287.0531  L=0.0065  h_trop=11000  h_strat=20000  rho0=1.225  P0=101325  T0=288.15  h0=0
      settings: SourceProductName=Aerospace Blockset
  Thrust : MATLAB Function  TreatAsAtomicUnit=on
  Thrust (N) : Outport
  Exit Pressure (Pa) : Outport  Port=2
  Exit Temperature (K) : Outport  Port=3
  Nozzle Exit Area (m²) : Outport  Port=4
  dmf (kg/s) : Outport  Port=5
  FN/del : Outport  Port=6
  wires:
  Thrust/4(Ae) -> Nozzle Exit Area (m²)/1
  Thrust/1(FN) -> Thrust (N)/1
  Thrust/3(Te) -> Exit Temperature (K)/1
  Thrust/2(Pe) -> Exit Pressure (Pa)/1
  To out (K)/1 -> Thrust/8(To2)
  Po out (Pa)/1 -> Thrust/7(Po2)
  Hot Heat Capacity Ratio/1 -> Thrust/9(gamma_h)
  Mass Flux out (kg/s)/1 -> Thrust/6(mass_flux)
  Mass Flux in (kg/s)/1 -> Thrust/5(mass_flux_0)
  ISA Atmosphere Model1/2 -> Thrust/2(a)
  Mach in/1 -> Thrust/1(Mo)
  Altitude (m)/1 -> ISA Atmosphere Model1/1
  ISA Atmosphere Model1/3 -> Thrust/3(Patm)
  ISA Atmosphere Model1/1 -> Thrust/4(Tatm)
  Thrust/5(dmf) -> dmf (kg/s)/1
  Thrust/6(FN_del) -> FN/del/1

== matlab function motorlib/Compressor/Compressor ==
  data: Po2 output; To2 output; mass_flux output; Po1 input; To1 input; m_air input; W output; gamma input; Cp input; PR input; eff input
function [Po2,To2,mass_flux,W] = Compressor(Po1,To1,m_air,gamma,Cp,PR,eff)
    Po2 = PR*Po1;   % total pressure out
    To2s = PR.^((gamma-1)/gamma) * To1;  % total isentropic temperature out
    To2 = (To2s-To1)/eff + To1; % total temperature out
    
    mass_flux = m_air; % mass flux out
   
    W=m_air*Cp*(To1-To2); % work used by the compressor

== matlab function motorlib/Thrust Meter/Thrust ==
  data: Mo input; a input; FN output; Patm input; Tatm input; mass_flux_0 input; mass_flux input; Po2 input; To2 input; Pe output; Te output; Ae output; gamma_h input
function [FN,Pe,Te,Ae] = Thrust(Mo,a,Patm,Tatm,mass_flux_0,mass_flux,Po2,To2,gamma_h)
    
    R = 287; % [J/kgK]

    % check if flow is choked
    choque = Po2/Patm;  
    PRsonico = (1 + (gamma_h-1)/2)^(gamma_h/(gamma_h-1));
    if choque>=PRsonico
      Pe=Po2/PRsonico;
      Te=To2/((PRsonico)^((gamma_h-1)/gamma_h));
    else
      Pe = Patm;
      Te = Tatm;
    end
    
    ue=sqrt(gamma_h*R*Te); % [m/s] exit speed
    Ae=(mass_flux*Te*R)/(Pe*ue); % [m^2] exit area for Mach 1
    
    uo = Mo*a;  % [m/s] inlet speed
    
    % specific Thurst
    FN = mass_flux*ue - mass_flux_0*uo + (Pe-Patm)*Ae;

== matlab function motorlib/Burner/Burner ==
  data: Po1 input; Po2 output; To2 output; To1 input; To2 input; mass_flux output; m_air input; gamma_c input; gamma_h input; Cp_c input; Cp_h input; PL input; eff input; PCI input
function [Po2,To2,mass_flux] = Burner(Po1,To1,To2,m_air,gamma_c,gamma_h,Cp_c,Cp_h,PL,eff,PCI)
    PR = 1 - PL;    % pressure ratio   
    Po2 = PR*Po1;
    
    f=(Cp_h*To2 - Cp_c*To1)/(eff*PCI + Cp_h*To2);
    
    m_f = m_air*f;
    mass_flux = m_air + m_f;

== matlab function motorlib/Turbine/Turbine ==
  data: Po1 input; To1 input; mass_flux input; W input; Po2 output; To2 output; gamma_h input; Cp_h input; eff input; mass_flux output
function [Po2,To2,mass_flux]  = Turbine(Po1,To1,mass_flux,W,gamma_h,Cp_h,eff)   
    To2 = W/(Cp_h*mass_flux) + To1; % real total temperature
    
    To2s = (To2-To1)/eff + To1; % isentropic total temperature
    
    PR = (To2s/To1).^(gamma_h/(gamma_h-1));   % pressure ratio
    Po2 = PR*Po1;   % total pressure

== matlab function motorlib/Nozzle/Nozzle ==
  data: Po1 input; Po2 output; To1 input; mass_flux input; gamma input; To2 output; mass_flux output; PL input
function [Po2,To2,mass_flux] = Nozzle(Po1,To1,mass_flux,gamma,PL)
    PR = 1-PL;
    
    Po2 = PR*Po1;
    To2 = To1;

== matlab function motorlib/Inlet/Inlet ==
  data: Mach input; Po output; P input; To output; T input; gamma input; PL input; m_air input; mass_flux output
function [Po,To,mass_flux] = Inlet(Mach,P,T,gamma,PL,m_air)
    % total pressure ratio inside the inlet
    PR = 1 - PL;
    
    % total pressure [Pa]
    Po = P*(1 + Mach.^2*(gamma-1)*0.5).^(gamma/(gamma-1));
    
    % total pressure with loss through the inlet [Pa]
    Po = PR * Po; 
    
    % total temperature [K]
    To = T*(1 + Mach.^2*(gamma-1)*0.5);
    
    mass_flux = m_air;

== matlab function motorlib/Bypass/Bypass ==
  data: Po1 input; To1 input; mass_flux input; gamma input; Po2 output; PL input; To2 output; mass_flux output
function [Po2,To2,mass_flux] = Bypass(Po1,To1,mass_flux,gamma,PL)
    PR = 1 - PL;
    Po2 = PR*Po1;
    To2 = To1*PR^((gamma-1)/gamma);

== matlab function motorlib/Fan/Fan ==
  data: Po1 input; To1 input; mass_flux input; gamma input; Cp input; PR input; eff input; B input; Po2 output; To2 output; mass_flux_bp output; mass_flux_core output; W output
function [Po2,To2,mass_flux_bp,mass_flux_core,W] = Fan(Po1,To1,mass_flux,gamma,Cp,PR,eff,B)
    Po2 = PR*Po1;   % total pressure out
    To2s = PR^((gamma-1)/gamma) * To1;  % total isentropic temperature out
    To2 = (To2s-To1)/eff + To1; % total temperature out
    
    W=mass_flux*Cp*(To1-To2); % work used by the compressor
    
    mass_flux_core = mass_flux/(1+B); % mass flux out to the core
    mass_flux_bp = mass_flux - mass_flux_core; % mass flux out to bypass

== matlab function motorlib/Total Plot ==
  data: P input; T input
function TotalPlot(P,T)
    figure    
    if(P)
        subplot(2,1,1)
        plot([P(1);P])
        title('Total Pressure through Engine (Pa)')
        xlabel('Engine Stages')
        ylabel('Total Pressure (Pa)')
        grid on
    else
        subplot(2,1,1,'replace')
    end
       
    if(T)
        subplot(2,1,2);
        plot([T(1);T])
        title('Total Temperauture through Engine (K)')
        xlabel('Engine Stages')
        ylabel('Total Temperature (K)')
        grid on
    else
        subplot(2,1,2,'replace')
    end

== matlab function motorlib/Turbojet Matching/Turbojet Matching ==
  data: M0 input; PRd output; PRc output; Me input; To2 input; To4 input; PRb input; PRn input; A1_A2 input; A2_A4 input; Ae_A4 input; gamma input; PRb output; PRt output; PRn output
function [PRd,PRc,PRb,PRt,PRn] = TurbojetMaching(M0,Me,To2,To4,PRb,PRn,A1_A2,A2_A4,Ae_A4,gamma)
    R = 287;             % [J/kgK]

    TRd = 1;            % diffuser temperature ratio
    TRb = PRb^((gamma-1)/gamma); % burner temperature ratio
    TRn = PRb^((gamma-1)/gamma); % nozzle temperature ratio
    theta =  To4/To2;   % turbine/compressore temperature ratio
    
    % mass flux matching fully expanded nozzle/turbine entry
    TRt = (1/Ae_A4)^(2*(gamma-1)/(gamma+1));
    PRt = TRt^(gamma/(gamma-1));

    % power matching compressor/turbine
    TRc = 1 + theta * (1 - TRt);
    PRc = TRc^(gamma/(gamma-1));

    % mass flux matching compressor/turbine entry
    % f<<1
    fM2 = PRc*PRb/(theta^0.5) * 1/A2_A4;

    % mass flux matching inlet/compressor
    expoente = (gamma+1)/(gamma-1);
    numerador = 2/(gamma+1) * (1 + (gamma-1)/2 * M0^2);
    fM0 = sqrt(M0^2/numerador^expoente);

    % diffuser pressure ratio
    PRd = A1_A2 * fM0/fM2;

    % total pressure ratio exit/ambient
    Poe_Poa = PRd*PRc*PRb*PRt*PRn;

    % static pressure ratio exit/ambient
    Pe_Pa = Poe_Poa * ((1 + (gamma-1)/2 * M0^2)/(1 + (gamma-1)/2 * Me^2))^(gamma/(gamma-1));

    % total temperature ratio exit/ambient
    Toe_Toa = theta * TRt;

    % static pressure ratio exit/ambient
    Te_Ta = Toe_Toa * (1 + (gamma-1)/2 * M0^2)/(1 + (gamma-1)/2 * Me^2);

    % velocity ratio
    ue_u0 = Me/M0 * Te_Ta^0.5;

    % entry/exit area ratio
    Ae_A1 = Ae_A4 * 1/A2_A4 * 1/A1_A2;

    % thrust family
    FN_A1Pa = gamma*M0^2 * (ue_u0 - 1) + Ae_A1 * (Pe_Pa - 1);

    PR = [1,PRd,PRc,PRb,PRt,PRn]';
    TR = [1,TRd,TRc,TRb,TRt,TRn]';

    Poi_Poa = PR;
    Toi_Toa = TR;
    
    for i=2:length(PR)
        Poi_Poa(i) = Poi_Poa(i-1) * PR(i);
        if(i==4)
            Toi_Toa(i) = theta;
        else    
            Toi_Toa(i) = Toi_Toa(i-1) * TR(i);
        end
    end
    
    figure    
    subplot(2,1,1)
    plot(Poi_Poa)
    title('Total Pressure Ratio')
    xlabel('Engine Stages')
    ylabel('Poi/Poa')
    grid on
    
    subplot(2,1,2)
    plot(Toi_Toa)
    grid on
    title('Total Temperature Ratio')
    xlabel('Engine Stages')
    ylabel('Toi/Toa')

== matlab function motorlib/Design Inlet/Inlet ==
  data: Mach input; Po output; P input; To output; T input; gamma input; PR input; m_air input; mass_flux output
function [Po,To,mass_flux] = Inlet(Mach,P,T,gamma,PR,m_air)   
    % total pressure [Pa]
    Po = P*(1 + Mach^2*(gamma-1)*0.5)^(gamma/(gamma-1));
    
    % total pressure with loss through the inlet [Pa]
    Po = PR * Po; 
    
    % total temperature [K]
    To = T*(1 + Mach^2*(gamma-1)*0.5);
    
    mass_flux = m_air;

== matlab function motorlib/Design Compressor/Compressor ==
  data: Po2 output; To2 output; mass_flux output; Po1 input; To1 input; m_air input; gamma input; Cp input; PR input; eff input
function [Po2,To2,mass_flux] = Compressor(Po1,To1,m_air,gamma,Cp,PR,eff)
    Po2 = PR*Po1;   % total pressure out
    To2s = PR^((gamma-1)/gamma) * To1;  % total isentropic temperature out
    To2 = (To2s-To1)/eff + To1; % total temperature out
    
    mass_flux = m_air; % mass flux out

== matlab function motorlib/Design Burner/Burner ==
  data: Po1 input; Po2 output; To2 output; To1 input; To2 input; mass_flux output; m_air input; gamma_c input; gamma_h input; Cp_c input; Cp_h input; PR input; eff input; PCI input
function [Po2,To2,mass_flux] = Burner(Po1,To1,To2,m_air,gamma_c,gamma_h,Cp_c,Cp_h,PR,eff,PCI)
    Po2 = PR*Po1;
    
    f=(Cp_h*To2 - Cp_c*To1)/(eff*PCI + Cp_h*To2);
    
    m_f = m_air*f;
    mass_flux = m_air + m_f;

== matlab function motorlib/Design Turbine/Turbine ==
  data: Po1 input; To1 input; mass_flux input; PR input; Po2 output; To2 output; gamma input; mass_flux output; eff input
function [Po2,To2,mass_flux]  = Turbine(Po1,To1,mass_flux,PR,gamma,eff)   
    Po2 = PR*Po1;   % total pressure   
    To2s = PR^((gamma-1)/gamma) * To1
    To2 = (To2s - To1)*eff + To1

== matlab function motorlib/Design Nozzle/Nozzle ==
  data: Po1 input; Po2 output; To1 input; mass_flux input; gamma input; To2 output; mass_flux output; PR input
function [Po2,To2,mass_flux] = Nozzle(Po1,To1,mass_flux,gamma,PR)
    Po2 = PR*Po1;
    To2 = To1;

== matlab function motorlib/Turbofan Matching/Turbofan Matching ==
  data: M0 input; PRd output; PRf output; PRhpc output; Me input; To2 input; To4 input; PRb input; PRn input; A7_A3 input; A5_A2 input; A4_A2 input; A2_A2f input; B input; gamma input; PRb output; PRhpt output; PRlpt output; PRn output; PRbp output
function [PRd,PRf,PRhpc,PRb,PRhpt,PRlpt,PRn,PRbp] = TurbofanMaching(M0,Me,To2,To4,PRb,PRn,A7_A3,A5_A2,A4_A2,A2_A2f,B,gamma)
    R = 287;            % [J/kgK]
    
    PRbp = 1;           % bypass pressure ratio
    TRbp = 1;           % bypass temperature ratio
    PRd = 1;            % diffuser pressure ratio
    TRd = 1;            % diffuser temperature ratio
    TRb = PRb^((gamma-1)/gamma); % burner temperature ratio
    TRn = PRb^((gamma-1)/gamma); % nozzle temperature ratio
    theta =  To4/To2;   % turbine/compressore temperature ratio
    
    %% mass flux matching HPC/HPT
    fM2 = sqrt(Me^2/(((gamma+1)/(gamma-1)) ^ ((2 / (gamma+1)) * (1 + (gamma-1)/2 * Me^2))))
    PRhpc = fM2/PRb * sqrt(To4/To2) * 1/A4_A2;
    TRhpc = PRhpc^((gamma-1)/gamma);

    %% power matching HPC/HPT
    TRhpt = ((-TRhpc +1) * To2 / To4) + 1;
    PRhpt = TRhpt^(gamma/(gamma-1));

    To5 = TRhpt * To4;
    
    %% mass flux matching HPC/LPT
    PRlpt = fM2 * sqrt(To5/To2) * 1/A5_A2 / (PRhpc * PRb);
    TRlpt = PRlpt^((gamma-1)/gamma);
    
    %% power matching Fan/LPT
    TRf = To5*(1-TRlpt)/((1+B)*To2) + 1;
    PRf = TRf^(gamma/(gamma-1));
    
    %% mass flux matching Fan/HPC
    fM2fan = (1 + B) * PRf * A2_A2f * sqrt(1/TRf) * fM2;
    
    %% mass flux matching Inlet/Fan
    fM0 = sqrt(M0^2/(((gamma+1)/(gamma-1)) ^ ((2 / (gamma+1)) * (1 + (gamma-1)/2 * M0^2))))
    A2_A1f = fM0/(PRd * fM2fan);
    
    %% mass flux matching Fan/Bypass Nozzle
    fM3 = TRbp ^ ((gamma + 1)/ 2 * (gamma - 1)) * A7_A3;
    
    %% mass flux matching HPT/Nozzle
    A4e = (TRhpt * TRlpt) ^ ((gamma + 1)/ 2 * (gamma - 1));
    
    %% 
    
    % total pressure ratio exit/ambient
    Poe_Poa = PRd*PRf*PRhpc*PRb*PRhpt*PRlpt*PRn;
    Pobp_Poa = PRd*PRf*PRbp;
 
    % static pressure ratio exit/ambient
    Pe_Pa = Poe_Poa * ((1 + (gamma-1)/2 * M0^2)/(1 + (gamma-1)/2 * Me^2))^(gamma/(gamma-1));

    % total temperature ratio exit/ambient
    Toe_Toa = theta * TRhpt;

    % static pressure ratio exit/ambient
    Te_Ta = Toe_Toa * (1 + (gamma-1)/2 * M0^2)/(1 + (gamma-1)/2 * Me^2);
 
%     % velocity ratio
%     ue_u0 = Me/M0 * Te_Ta^0.5;
% 
%     % entry/exit area ratio
%     Ae_A1 = Ae_A4 * 1/A2_A4 * 1/A1_A2;
% 
%     % thrust family
%     FN_A1Pa = gamma*M0^2 * (ue_u0 - 1) + Ae_A1 * (Pe_Pa - 1);

    PR = [1,PRd,PRf,PRhpc,PRb,PRhpt,PRlpt,PRn]';
    PR_ = [1,PRd,PRf,PRbp]';
    TR = [1,TRd,TRf,TRhpc,TRb,TRhpt,TRlpt,TRn]';
    TR_ = [1,TRd,TRf,TRbp]';

    Poi_Poa = PR;
    Poi_Poa_bp = PR_;
    Toi_Toa = TR;
    Toi_Toa_bp = TR_;
    
    for i=2:length(PR)
        Poi_Poa(i) = Poi_Poa(i-1) * PR(i);
        if(i==4)
            Toi_Toa(i) = theta;
        else    
            Toi_Toa(i) = Toi_Toa(i-1) * TR(i);
        end
    end
    
    figure    
    subplot(2,1,1)
    plot(Poi_Poa)
    hold on
    plot([1,2,3,4.5],Poi_Poa_bp,'--')
    title('Total Pressure Ratio')
    xlabel('Engine Stages')
    ylabel('Poi/Poa')
    grid on
    
    subplot(2,1,2)
    plot(Toi_Toa)
    hold on
    plot([1,2,3,4.5],Toi_Toa_bp,'--')
    grid on
    title('Total Temperature Ratio')
    xlabel('Engine Stages')
    ylabel('Toi/Toa')

== matlab function motorlib/Design Fan/Fan ==
  data: Po1 input; To1 input; mass_flux input; gamma input; Cp input; PR input; eff input; B input; Po2 output; To2 output; mass_flux_bp output; mass_flux_core output
function [Po2,To2,mass_flux_bp,mass_flux_core] = Fan(Po1,To1,mass_flux,gamma,Cp,PR,eff,B)
    Po2 = PR*Po1;   % total pressure out
    To2s = PR^((gamma-1)/gamma) * To1;  % total isentropic temperature out
    To2 = (To2s-To1)/eff + To1; % total temperature out
    
    W=mass_flux*Cp*(To1-To2); % work used by the compressor
    
    mass_flux_core = mass_flux/(1+B); % mass flux out to the core
    mass_flux_bp = mass_flux - mass_flux_core; % mass flux out to bypass

== matlab function motorlib/Design Bypass/Bypass ==
  data: Po1 input; To1 input; mass_flux input; gamma input; Po2 output; PR input; To2 output; mass_flux output
function [Po2,To2,mass_flux] = Bypass(Po1,To1,mass_flux,gamma,PR)
    
    Po2 = PR*Po1;
    To2 = To1*PR^((gamma-1)/gamma);

== matlab function motorlib/Aircraft/Aircraft ==
  data: W input; Sg output; S input; CL input; CD input; Fn input; dmf input; t input; M input; Sc output; mf output; p input; rho input; D_del output
function [Sg,Sc,mf,D_del] = Aircraft(W,S,CL,CD,Fn,dmf,t,M,p,rho)
    g = 9.81;   % [m/s^2]  gravity acceleration
    mu = 0.02;  %          fricction coefficient
    p_std = 101.3e3; % [Pa] standard pressure
    gamma = 1.4;    % specific heat ratio
    
    W = W*g;    % [N] weight
    t = t*3600; % [s] flight duration
    
    Vstall = sqrt(W/(CL*rho*S));    % [m/s] stall velocity
    Vlo = 1.2*Vstall;                   % [m/s] lift-off velocity
    
    a = g*(Fn - mu*W)/W;    % [m/s^2] mean acceleration 
    Sg = Vlo^2/(2*a);       % [m] ground-roll distance
    
    % ?????????????????????? Vlo or Vle = 1/2Vstall ?
    dt = Vlo/(2*a);         % [s] ground-roll time
    
    TSFC = dmf/Fn;
    mf = dmf*(dt+t);    % [kg]   fuel mass consumption per flight
    
    W1 = W;
    W2 = W1 - mf*g;
   
    % [m] level flight distance
    Sc = (2/(TSFC*g))*sqrt(2*CL/(S*rho*CD))*(sqrt(W1)-sqrt(W2));
      
    del = p/p_std;
    
    % power required
    M = 0:0.02:0.9;
    D_del = gamma*0.5*p_std*CL*M.^2*S;
    
    % power available
    Fn_del = Fn/del;

== matlab function motorlib/Turbojet/Thrust Meter1/Thrust ==
  data: Mo input; a input; FN output; Patm input; Tatm input; mass_flux_0 input; mass_flux input; Po2 input; To2 input; Pe output; Te output; Ae output; gamma_h input; dmf output; FN_del output
function [FN,Pe,Te,Ae,dmf,FN_del] = Thrust(Mo,a,Patm,Tatm,mass_flux_0,mass_flux,Po2,To2,gamma_h)
    
    R = 287; % [J/kgK]

    % check if flow is choked
    choque = Po2/Patm;  
    PRsonico = (1 + (gamma_h-1)/2)^(gamma_h/(gamma_h-1));
    if choque>=PRsonico
      Pe=Po2/PRsonico;
      Te=To2/((PRsonico)^((gamma_h-1)/gamma_h));
    else
      Pe = Patm;
      Te = Tatm;
    end
    
    ue=sqrt(gamma_h*R*Te); % [m/s] exit speed
    Ae=(mass_flux*Te*R)/(Pe*ue); % [m^2] exit area for Mach 1
           
    uo = Mo*a;  % [m/s] inlet speed
    
    % specific Thurst
    FN = mass_flux*ue - mass_flux_0*uo + (Pe-Patm)*Ae;
    
    dmf = (mass_flux-mass_flux_0);
    
    del = Patm/101.3e3;
    FN_del = FN/del;

== matlab function motorlib/Concorde/Aircraft ==
  data: W input; Sg output; S input; CL input; CD input; Fn input; dmf input; t input; M input; Sc output; mf output; p input; rho input; D_del output
function [Sg,Sc,mf,D_del] = Aircraft(W,S,CL,CD,Fn,dmf,t,M,p,rho)
    g = 9.81;   % [m/s^2]  gravity acceleration
    mu = 0.02;  %          fricction coefficient
    p_std = 101.3e3; % [Pa] standard pressure
    gamma = 1.4;    % specific heat ratio
    
    W = W*g;    % [N] weight
    t = t*3600; % [s] flight duration
    
    Vstall = sqrt(W/(CL*rho*S));    % [m/s] stall velocity
    Vlo = 1.2*Vstall;                   % [m/s] lift-off velocity
    
    a = g*(Fn - mu*W)/W;    % [m/s^2] mean acceleration 
    Sg = Vlo^2/(2*a);       % [m] ground-roll distance
    
    % ?????????????????????? Vlo or Vle = 1/2Vstall ?
    dt = Vlo/(2*a);         % [s] ground-roll time
    
    TSFC = dmf/Fn;
    mf = dmf*(dt+t);    % [kg]   fuel mass consumption per flight
    
    W1 = W;
    W2 = W1 - mf*g;
   
    % [m] level flight distance
    Sc = (2/(TSFC*g))*sqrt(2*CL/(S*rho*CD))*(sqrt(W1)-sqrt(W2));
      
    del = p/p_std;
    
    % power required
    M = 0:0.02:0.9;
    D_del = gamma*0.5*p_std*CL*M.^2*S;
    
    % power available
    Fn_del = Fn/del;

== matlab function motorlib/SR-71 BlackBird/Aircraft ==
  data: W input; Sg output; S input; CL input; CD input; Fn input; dmf input; t input; M input; Sc output; mf output; p input; rho input; D_del output
function [Sg,Sc,mf,D_del] = Aircraft(W,S,CL,CD,Fn,dmf,t,M,p,rho)
    g = 9.81;   % [m/s^2]  gravity acceleration
    mu = 0.02;  %          fricction coefficient
    p_std = 101.3e3; % [Pa] standard pressure
    gamma = 1.4;    % specific heat ratio
    
    W = W*g;    % [N] weight
    t = t*3600; % [s] flight duration
    
    Vstall = sqrt(W/(0.5*CL*rho*S))    % [m/s] stall velocity
    Vlo = 1.2*Vstall                   % [m/s] lift-off velocity
    
    a = g*(Fn - mu*W)/W   % [m/s^2] mean acceleration 
    Sg = Vlo^2/(2*a)       % [m] ground-roll distance
    
    % ?????????????????????? Vlo or Vle = 1/2Vstall ?
    dt = Vlo/(2*a)         % [s] ground-roll time
    
    TSFC = dmf/Fn;
    mf = dmf*(dt+t);    % [kg]   fuel mass consumption per flight
    
    
   
    % [m] level flight distance
    Sc = M*340/g * 1/TSFC * CL/CD * t*(16/3 * CD/(pi*0.95*16.94^2/S))^0.5;
      
    del = p/p_std;
    
    % power required
    M = 0:0.02:0.9;
    D_del = gamma*0.5*p_std*CL*M.^2*S;
    
    % power available
    Fn_del = Fn/del;

== matlab function motorlib/Bombardier 300/Aircraft ==
  data: W input; Sg output; S input; CL input; CD input; Fn input; dmf input; Wf input; M input; Sc output; mf output; p input; rho input; D_del output
function [Sg,Sc,mf,D_del] = Aircraft(W,S,CL,CD,Fn,dmf,Wf,M,p,rho)
    g = 9.81;   % [m/s^2]  gravity acceleration
    mu = 0.02;  %          fricction coefficient
    p_std = 101.3e3; % [Pa] standard pressure
    gamma = 1.4;    % specific heat ratio
    
    W = (W+Wf)*g;    % [N] weight
   
    Vstall = sqrt(W/(0.5*CL*rho*S));    % [m/s] stall velocity
    Vlo = Vstall*1.2;                   % [m/s] lift-off velocity
    
    a = g*(Fn - mu*W)/W;    % [m/s^2] mean acceleration 
    Sg = Vlo^2/(2*a);       % [m] ground-roll distance
    
    dt = Vlo/(2*a)        % [s] ground-roll time
    
    t = Wf/dmf
    Sc = t*(M*340)
    mf=Wf
    
    TSFC = dmf/Fn
    Sc = M*340/g * 1/TSFC * CL/CD * log((W+Wf)/W)
    
    
    % [m] level flight distance
    %Sc = (2/(TSFC*g))*sqrt(2*CL/(S*rho*CD))*(sqrt(W)-sqrt(W-Wf))
    %t = Sc/(M*340)
    
    %mf = dmf*dt
    %mf = dmf*(dt+t)    % [kg]   fuel mass consumption per flight
   
    del = p/p_std;
    
    % power required
    M = 0:0.02:0.9;
    D_del = gamma*0.5*p_std*CL*M.^2*S;
    
    % power available
    Fn_del = Fn/del;
